simulink model "TP2"  (R2015a)
settings: Solver=ode3  StartTime=0.0  StopTime=inf  FixedStep=0.05  RelTol=1e-3
undefined symbols (not defined in the file): serial
libraries: simulink x5, instrumentlib x3
settings Model: Creator=nico  LastModifiedBy=dani
settings DebuggingCC: UnderspecifiedInitializationDetection=Classic  MergeDetectMultiDrivingBlocksExec=none  SolverPrmCheckMsg=warning

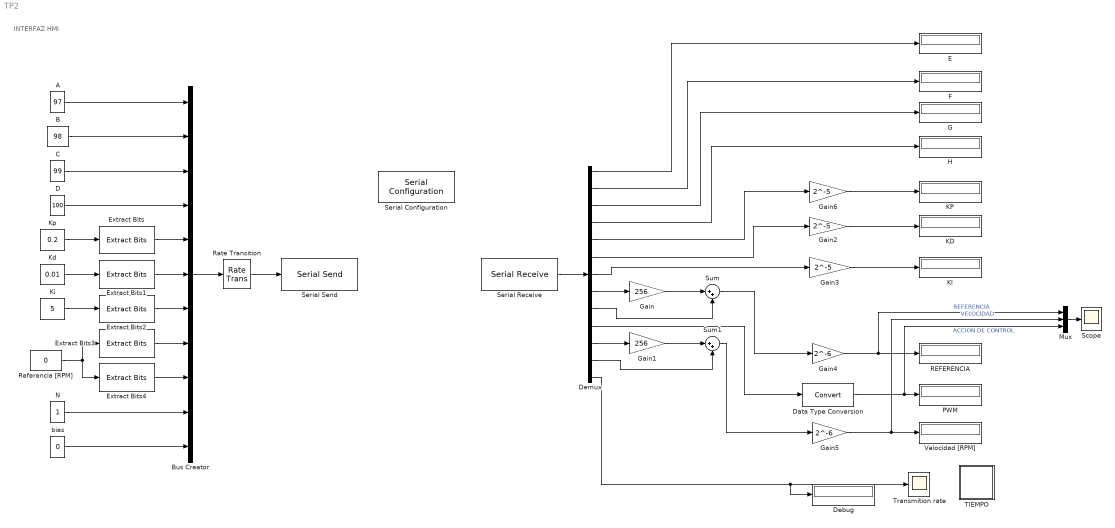
== system TP2 ==
  note: INTERFAZ HMI
  A : Constant  Value=97  OutDataTypeStr=uint8  SampleTime=1
  B : Constant  Value=98  OutDataTypeStr=uint8  SampleTime=1
  Bus Creator : BusCreator  Inputs=11
  C : Constant  Value=99  OutDataTypeStr=uint8  SampleTime=1
  D : Constant  Value=100  OutDataTypeStr=uint8  SampleTime=1
  Data Type Conversion : DataTypeConversion
  "Debug " : Display
  Demux : Demux  Outputs=13
  E : Display
  Extract Bits : simulink/Logic and Bit Operations/Extract Bits  bitsToExtract=Range starting with most significant bit  numBits=8  bitIdxRange=[0 7]  outScalingMode=Treat bit field as an integer
  Extract Bits1 : simulink/Logic and Bit Operations/Extract Bits  bitsToExtract=Range starting with most significant bit  numBits=8  bitIdxRange=[0 7]  outScalingMode=Treat bit field as an integer
  Extract Bits2 : simulink/Logic and Bit Operations/Extract Bits  bitsToExtract=Range starting with most significant bit  numBits=8  bitIdxRange=[0 7]  outScalingMode=Treat bit field as an integer
  Extract Bits3 : simulink/Logic and Bit Operations/Extract Bits  bitsToExtract=Upper half  numBits=8  bitIdxRange=[0 7]  outScalingMode=Treat bit field as an integer
  Extract Bits4 : simulink/Logic and Bit Operations/Extract Bits  bitsToExtract=Lower half  numBits=8  bitIdxRange=[0 7]  outScalingMode=Treat bit field as an integer
  F : Display
  G : Display
  Gain : Gain  Gain=256
  Gain1 : Gain  Gain=256
  Gain2 : Gain  Gain=2^-5
  Gain3 : Gain  Gain=2^-5
  Gain4 : Gain  Gain=2^-6
  Gain5 : Gain  Gain=2^-6
  Gain6 : Gain  Gain=2^-5
  H : Display
  KD : Display
  KI : Display
  KP : Display
  Kd : Constant  Value=0.01  OutDataTypeStr=fixdt(0,8,5)  SampleTime=1
  Ki : Constant  Value=5  OutDataTypeStr=fixdt(0,8,5)  SampleTime=1
  Kp : Constant  Value=0.2  OutDataTypeStr=fixdt(0,8,5, 'DataTypeOverride', 'Off')  SampleTime=1
  Mux : Mux  Inputs=3
  N : Constant  OutDataTypeStr=uint8  SampleTime=1
  PWM : Display
  REFERENCIA : Display
      settings: Decimation=3
  Rate Transition : RateTransition  Integrity=off  OutPortSampleTimeOpt=Inherit
  Referencia [RPM] : Constant  Value=0  OutDataTypeStr=fixdt(0,16,6)  SampleTime=1
  Scope : Scope
      settings: ShowLegends=on  TimeRange=20  YMin=0  YMax=300
  Serial Configuration : instrumentlib/Serial Configuration  Priority=-200000  ComPortMenu=<Please select a port...>  ComPort=COM4  ObjConstructor=serial('COM4');  BaudRate=9600  DataBits=8  Parity=none  StopBits=1  FlowControl=none  Timeout=20  ByteOrder=LittleEndian
  Serial Receive : instrumentlib/Serial Receive  ComPortMenu=COM4  ComPort=COM4  ObjConstructor=serial('COM4');  Terminator=<none>  DataSize="[13   1]"  DataType=uint8  EnableBlockingMode=on  ActionDataUnavailable=Output last received value  CustomValue=-1  SampleTime=0.1
  Serial Send : instrumentlib/Serial Send  ComPortMenu=<Please select a port...>  ComPort=COM4  ObjConstructor=serial('COM4');  Terminator=<none>  EnableBlockingMode=on
  Sum : Sum  Inputs=|++
  Sum1 : Sum  Inputs=|++
  TIEMPO : Subsystem  DialogController=hmiCreateDDGDialog  IsWebBlock=on  mask(MathWorksWebBlock){webBlockId=49241c16-f6af-4385-9617-47093c5dfdcb, webBlockType=lamp, ShowInLibBrowser=on, ShowInitialText=on, HMISrcModelName=TP2}
      mask prompts: webBlockType "WebBlock Type"; HMISrcModelName "Source Model"
      mask Help: helpview([docroot '/mapfiles/simulink.map'], 'hmi_lamp')
      mask Display:
      | if strcmp(get_param(bdroot(gcb),'BlockDiagramType'), 'library')
      |     image([(matlabroot) '/toolbox/simulink/hmi/icons/Lamp.png']);
      | end
  Transmition rate : Scope
      settings: YMin=100  YMax=100
  Velocidad [RPM] : Display
  bias : Constant  Value=0  OutDataTypeStr=uint8  SampleTime=1
  wires:
  A/1 -> Bus Creator/1
  Serial Receive/1 -> Demux/1
  Demux/1 -> E/1
  B/1 -> Bus Creator/2
  Demux/2 -> F/1
  Bus Creator/1 -> Rate Transition/1
  Demux/4 -> H/1
  Demux/3 -> G/1
  Gain/1 -> Sum/1
  Demux/8 -> Gain/1
  Demux/9 -> Sum/2
  Demux/10 -> Data Type Conversion/1
  Demux/11 -> Gain1/1
  Demux/12 -> Sum1/2
  Gain1/1 -> Sum1/1
  C/1 -> Bus Creator/3
  D/1 -> Bus Creator/4
  Referencia [RPM]/1 -> Extract Bits3/1, Extract Bits4/1
  N/1 -> Bus Creator/10
  Gain2/1 -> KD/1
  Demux/6 -> Gain2/1
  Gain3/1 -> KI/1
  Demux/7 -> Gain3/1
  Sum/1 -> Gain4/1
  Gain5/1 -> Mux/2, Velocidad [RPM]/1  "VELOCIDAD"
  Sum1/1 -> Gain5/1
  Gain4/1 -> Mux/1, REFERENCIA/1  "REFERENCIA"
  Rate Transition/1 -> Serial Send/1
  bias/1 -> Bus Creator/11
  Gain6/1 -> KP/1
  Demux/5 -> Gain6/1
  Kp/1 -> Extract Bits/1
  Kd/1 -> Extract Bits1/1
  Extract Bits/1 -> Bus Creator/5
  Extract Bits2/1 -> Bus Creator/7
  Extract Bits1/1 -> Bus Creator/6
  Ki/1 -> Extract Bits2/1
  Extract Bits3/1 -> Bus Creator/8
  Extract Bits4/1 -> Bus Creator/9
  Mux/1 -> Scope/1
  Data Type Conversion/1 -> Mux/3, PWM/1  "ACCION DE CONTROL"
  Demux/13 -> "Debug "/1, Transmition rate/1

== system TP2/TIEMPO ==
